simulink model "simulacion"  (R2019a)
settings: Solver=VariableStepAuto  StartTime=0.0  StopTime=20  RelTol=1e-3
libraries: cstblocks x4
settings Model: Creator=Juan P Velandia  LastModifiedBy=Juan P Velandia

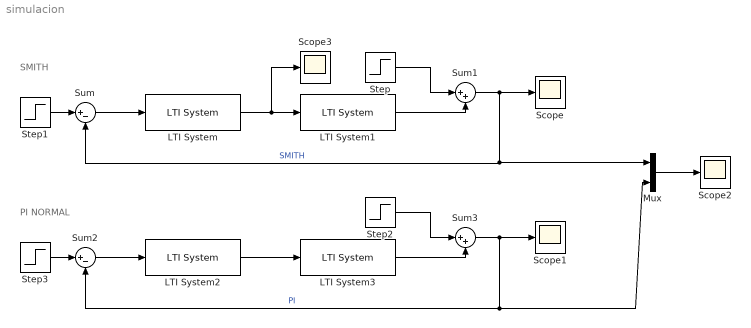
== system simulacion ==
  note: SMITH
  note: PI NORMAL
  LTI System : cstblocks/LTI System  sys=ceq  IC=[]
  LTI System1 : cstblocks/LTI System  sys=P  IC=[]
  LTI System2 : cstblocks/LTI System  sys=PI  IC=[]
  LTI System3 : cstblocks/LTI System  sys=P  IC=[]
  Mux : Mux  Inputs=2
  Scope{,1..3} (4 alike) : Scope
  Step : Step  Time=10  After=0.5  SampleTime=0
  Step1 : Step  Time=0  SampleTime=0
  Step2 : Step  Time=10  After=0.5  SampleTime=0
  Step3 : Step  Time=0  SampleTime=0
  Sum : Sum  Inputs=|+-
  Sum1 : Sum  Inputs=|++
  Sum2 : Sum  Inputs=|+-
  Sum3 : Sum  Inputs=|++
  wires:
  Sum/1 -> LTI System/1
  LTI System/1 -> Scope3/1, LTI System1/1
  Step1/1 -> Sum/1
  LTI System1/1 -> Sum1/2
  Step/1 -> Sum1/1
  Sum1/1 -> Scope/1, Mux/1, Sum/2  "SMITH"
  Sum2/1 -> LTI System2/1
  Step3/1 -> Sum2/1
  Sum3/1 -> Sum2/2, Mux/2, Scope1/1  "PI"
  Step2/1 -> Sum3/1
  LTI System2/1 -> LTI System3/1
  LTI System3/1 -> Sum3/2
  Mux/1 -> Scope2/1
